simulink model "gnc_simplified"  (R2025b)
settings: Solver=ode2  StartTime=0.0  StopTime=inf  FixedStep=1/100  RelTol=1e-3
undefined symbols (not defined in the file or in its folder): DiscIntNeverNeededParam, dspblkCoreblockFVToolHelper, gcbh
libraries: simulink x5, eeGeneralControl x5
(part 2 of 4)

== system gnc_simplified/INDI/Thrust ==
  note: float32 delta_t
      | float32 t_m
      | float32 t_c
  note: Current thrust
      | lever in [-1,1]
  note: Incremental thrust
      | command in [-1,1]
  note: Total thrust
      | command in [0,1]
  thr_inc : Inport  OutDataTypeStr=single  PortDimensions=1
  act_m : Inport  Port=2  OutDataTypeStr=single  PortDimensions=4
  Bias : Bias  Bias=-1  SaturateOnIntegerOverflow=off
  Bias1 : Bias  Bias=0.5  SaturateOnIntegerOverflow=off
  Constant : Constant  OutDataTypeStr=single
  Constant1 : Constant  Value=-1  OutDataTypeStr=single
  Gain : Gain  Gain=2
  Gain1 : Gain  Gain=0.5
  Gain2 : Gain  Gain=0.5
  Limit_Increment : simulink/Discontinuities/Saturation Dynamic  OutMin=[]  OutMax=[]  OutDataTypeStr=Inherit: Same as second input  OutDataType=fixdt(1, 16)  OutScaling=2^-10  DoSatur=off
  Minus1 : Sum  Inputs=+-
  Minus2 : Sum  Inputs=+-
  Mux : Mux  Inputs=3
  Plus1 : Sum
  Scope : Scope  NumInputPorts=4
      settings: ActiveDisplayYMinimum=-2.22188  ActiveDisplayYMaximum=2.10921
  Selector1 : Selector  InputPortWidth=4  IndexOptions=Index vector (dialog)  Indices=4  OutputSizes=1
  thr_moni : Outport  OutDataTypeStr=single  PortDimensions=3
  thr : Outport  Port=2  OutDataTypeStr=single  PortDimensions=1
  inc_moni : Outport  Port=3
  wires:
  Mux/1 -> thr_moni/1
  Bias/1 -> Scope/1, Mux/2, Minus1/2, Minus2/2, Scope/3, Plus1/2
  Gain/1 -> Bias/1
  Limit_Increment/1 -> Plus1/1, Gain2/1, Scope/2, Mux/1  "thr_inc"
  act_m/1 -> Selector1/1
  Selector1/1 -> Gain/1
  Plus1/1 -> Gain1/1
  Gain1/1 -> Bias1/1
  Bias1/1 -> Scope/4, Mux/3, thr/1
  Gain2/1 -> inc_moni/1
  Constant/1 -> Minus1/1
  thr_inc/1 -> Limit_Increment/2
  Minus1/1 -> Limit_Increment/1
  Minus2/1 -> Limit_Increment/3
  Constant1/1 -> Minus2/1

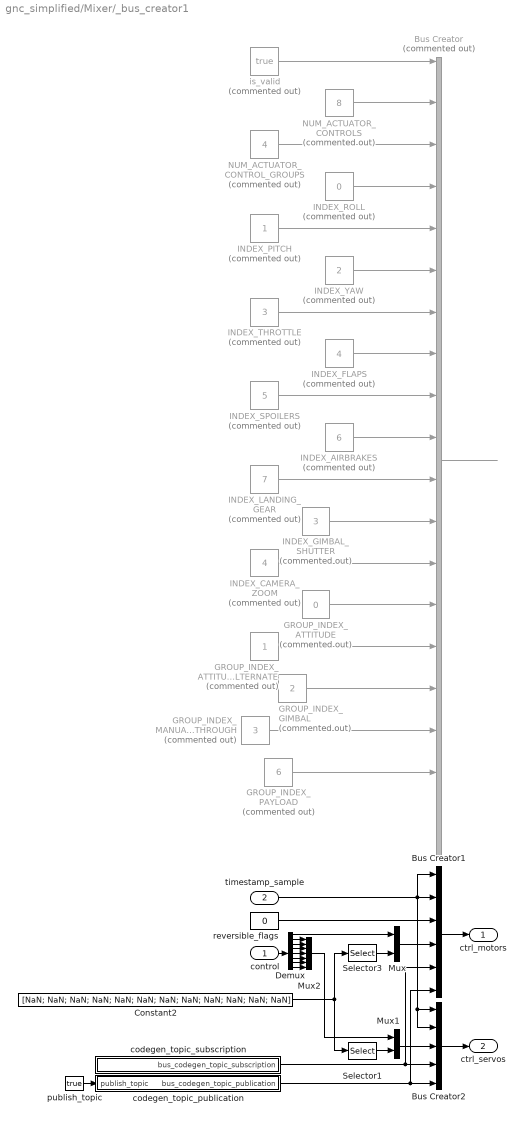
== system gnc_simplified/Mixer/_bus_creator1 ==
  control : Inport  OutDataTypeStr=single  PortDimensions=8
  timestamp_sample : Inport  Port=2  OutDataTypeStr=uint64  PortDimensions=1
  Bus Creator : BusCreator  Commented=on  Inputs=20  OutDataTypeStr=Bus:actuator_controls_0_bus
      settings: InheritFromInputs=off
  Bus Creator1 : BusCreator  Inputs=6  OutDataTypeStr=Bus: IFRCG_Bus_Topic_ActuatorMotors
      settings: InheritFromInputs=off
  Bus Creator2 : BusCreator  Inputs=5  OutDataTypeStr=Bus: IFRCG_Bus_Topic_ActuatorServos
      settings: InheritFromInputs=off
  Constant2 : Constant  Value=[NaN; NaN; NaN; NaN; NaN; NaN; NaN; NaN; NaN; NaN; NaN; NaN]  OutDataTypeStr=single
  Demux : Demux  Outputs=8
  GROUP_INDEX_ATTITUDE : Constant  Commented=on  Value=0  OutDataTypeStr=uint8
  GROUP_INDEX_ATTITUDE_ALTERNATE : Constant  Commented=on  OutDataTypeStr=uint8
  GROUP_INDEX_GIMBAL : Constant  Commented=on  Value=2  OutDataTypeStr=uint8
  GROUP_INDEX_MANUAL_PASSTHROUGH : Constant  Commented=on  Value=3  OutDataTypeStr=uint8
  GROUP_INDEX_PAYLOAD : Constant  Commented=on  Value=6  OutDataTypeStr=uint8
  INDEX_AIRBRAKES : Constant  Commented=on  Value=6  OutDataTypeStr=uint8
  INDEX_CAMERA_ZOOM : Constant  Commented=on  Value=4  OutDataTypeStr=uint8
  INDEX_FLAPS : Constant  Commented=on  Value=4  OutDataTypeStr=uint8
  INDEX_GIMBAL_SHUTTER : Constant  Commented=on  Value=3  OutDataTypeStr=uint8
  INDEX_LANDING_GEAR : Constant  Commented=on  Value=7  OutDataTypeStr=uint8
  INDEX_PITCH : Constant  Commented=on  OutDataTypeStr=uint8
  INDEX_ROLL : Constant  Commented=on  Value=0  OutDataTypeStr=uint8
  INDEX_SPOILERS : Constant  Commented=on  Value=5  OutDataTypeStr=uint8
  INDEX_THROTTLE : Constant  Commented=on  Value=3  OutDataTypeStr=uint8
  INDEX_YAW : Constant  Commented=on  Value=2  OutDataTypeStr=uint8
  Mux : Mux  Inputs=2
  Mux1 : Mux  Inputs=2
  Mux2 : Mux  Inputs=7
  NUM_ACTUATOR_CONTROLS : Constant  Commented=on  Value=8  OutDataTypeStr=uint8
  NUM_ACTUATOR_CONTROL_GROUPS : Constant  Commented=on  Value=4  OutDataTypeStr=uint8
  Selector1 : Selector  InputPortWidth=12  IndexOptions=Index vector (dialog)  Indices=1  OutputSizes=1
  Selector3 : Selector  InputPortWidth=12  IndexOptions=Index vector (dialog)  Indices=1:11  OutputSizes=1
  codegen_topic_publication : Subsystem
  codegen_topic_subscription : Subsystem
  is_valid : Constant  Commented=on  Value=true  OutDataTypeStr=boolean
  publish_topic : Constant  Value=true  OutDataTypeStr=boolean
  reversible_flags : Constant  Value=0  OutDataTypeStr=uint16
  ctrl_motors : Outport  OutDataTypeStr=Bus: IFRCG_Bus_Topic_ActuatorMotors  VectorParamsAs1DForOutWhenUnconnected=off
  ctrl_servos : Outport  Port=2  OutDataTypeStr=Bus: IFRCG_Bus_Topic_ActuatorServos  VectorParamsAs1DForOutWhenUnconnected=off
  wires:
  Bus Creator/1 -> ?
  ? -> Bus Creator/20
  ? -> Bus Creator/19
  GROUP_INDEX_ATTITUDE_ALTERNATE/1 -> Bus Creator/15
  GROUP_INDEX_ATTITUDE/1 -> Bus Creator/14
  INDEX_LANDING_GEAR/1 -> Bus Creator/11
  INDEX_AIRBRAKES/1 -> Bus Creator/10
  INDEX_SPOILERS/1 -> Bus Creator/9
  INDEX_FLAPS/1 -> Bus Creator/8
  INDEX_THROTTLE/1 -> Bus Creator/7
  INDEX_YAW/1 -> Bus Creator/6
  INDEX_PITCH/1 -> Bus Creator/5
  INDEX_ROLL/1 -> Bus Creator/4
  NUM_ACTUATOR_CONTROL_GROUPS/1 -> Bus Creator/3
  NUM_ACTUATOR_CONTROLS/1 -> Bus Creator/2
  is_valid/1 -> Bus Creator/1
  INDEX_GIMBAL_SHUTTER/1 -> Bus Creator/12
  INDEX_CAMERA_ZOOM/1 -> Bus Creator/13
  GROUP_INDEX_GIMBAL/1 -> Bus Creator/16
  GROUP_INDEX_MANUAL_PASSTHROUGH/1 -> Bus Creator/17
  GROUP_INDEX_PAYLOAD/1 -> Bus Creator/18
  Bus Creator1/1 -> ctrl_motors/1
  Bus Creator2/1 -> ctrl_servos/1
  Mux1/1 -> Bus Creator2/3
  timestamp_sample/1 -> Bus Creator2/1, Bus Creator2/2, Bus Creator1/1, Bus Creator1/2
  reversible_flags/1 -> Bus Creator1/3
  publish_topic/1 -> codegen_topic_publication/1(publish_topic)
  codegen_topic_subscription/1(bus_codegen_topic_subscription) -> Bus Creator2/4, Bus Creator1/5
  codegen_topic_publication/1(bus_codegen_topic_publication) -> Bus Creator1/6, Bus Creator2/5
  Selector3/1 -> Mux/2
  Mux/1 -> Bus Creator1/4
  Demux/2 -> Mux2/1
  Demux/3 -> Mux2/2
  Demux/4 -> Mux2/3
  Demux/5 -> Mux2/4
  Demux/6 -> Mux2/5
  Demux/7 -> Mux2/6
  Demux/8 -> Mux2/7
  control/1 -> Demux/1
  Demux/1 -> Mux/1
  Mux2/1 -> Mux1/1
  Selector1/1 -> Mux1/2
  Constant2/1 -> Selector1/1, Selector3/1

== system gnc_simplified/Mixer/_bus_creator2 ==
  control : Inport  OutDataTypeStr=single  PortDimensions=8
  timestamp_sample : Inport  Port=2  OutDataTypeStr=double  PortDimensions=1
  Bus Creator : BusCreator  Inputs=20  OutDataTypeStr=Bus:actuator_controls_0_bus
      settings: InheritFromInputs=off
  GROUP_INDEX_ATTITUDE : Constant  Value=0  OutDataTypeStr=uint8
  GROUP_INDEX_ATTITUDE_ALTERNATE : Constant  OutDataTypeStr=uint8
  GROUP_INDEX_GIMBAL : Constant  Value=2  OutDataTypeStr=uint8
  GROUP_INDEX_MANUAL_PASSTHROUGH : Constant  Value=3  OutDataTypeStr=uint8
  GROUP_INDEX_PAYLOAD : Constant  Value=6  OutDataTypeStr=uint8
  INDEX_AIRBRAKES : Constant  Value=6  OutDataTypeStr=uint8
  INDEX_CAMERA_ZOOM : Constant  Value=4  OutDataTypeStr=uint8
  INDEX_FLAPS : Constant  Value=4  OutDataTypeStr=uint8
  INDEX_GIMBAL_SHUTTER : Constant  Value=3  OutDataTypeStr=uint8
  INDEX_LANDING_GEAR : Constant  Value=7  OutDataTypeStr=uint8
  INDEX_PITCH : Constant  OutDataTypeStr=uint8
  INDEX_ROLL : Constant  Value=0  OutDataTypeStr=uint8
  INDEX_SPOILERS : Constant  Value=5  OutDataTypeStr=uint8
  INDEX_THROTTLE : Constant  Value=3  OutDataTypeStr=uint8
  INDEX_YAW : Constant  Value=2  OutDataTypeStr=uint8
  NUM_ACTUATOR_CONTROLS : Constant  Value=8  OutDataTypeStr=uint8
  NUM_ACTUATOR_CONTROL_GROUPS : Constant  Value=4  OutDataTypeStr=uint8
  is_valid : Constant  Value=true  OutDataTypeStr=boolean
  actuator_controls : Outport  OutDataTypeStr=Bus: IFRCG_Bus_Topic_ActuatorControls1  VectorParamsAs1DForOutWhenUnconnected=off
  wires:
  INDEX_ROLL/1 -> Bus Creator/4
  INDEX_SPOILERS/1 -> Bus Creator/9
  is_valid/1 -> Bus Creator/1
  INDEX_CAMERA_ZOOM/1 -> Bus Creator/13
  control/1 -> Bus Creator/20
  GROUP_INDEX_ATTITUDE_ALTERNATE/1 -> Bus Creator/15
  GROUP_INDEX_GIMBAL/1 -> Bus Creator/16
  INDEX_GIMBAL_SHUTTER/1 -> Bus Creator/12
  INDEX_THROTTLE/1 -> Bus Creator/7
  GROUP_INDEX_ATTITUDE/1 -> Bus Creator/14
  Bus Creator/1 -> actuator_controls/1
  INDEX_PITCH/1 -> Bus Creator/5
  GROUP_INDEX_MANUAL_PASSTHROUGH/1 -> Bus Creator/17
  INDEX_FLAPS/1 -> Bus Creator/8
  INDEX_AIRBRAKES/1 -> Bus Creator/10
  NUM_ACTUATOR_CONTROLS/1 -> Bus Creator/2
  GROUP_INDEX_PAYLOAD/1 -> Bus Creator/18
  timestamp_sample/1 -> Bus Creator/19
  INDEX_YAW/1 -> Bus Creator/6
  NUM_ACTUATOR_CONTROL_GROUPS/1 -> Bus Creator/3
  INDEX_LANDING_GEAR/1 -> Bus Creator/11

== system gnc_simplified/Mixer/bus_generator ==
  In1 : Inport
  Bus Creator : BusCreator  Inputs=7  OutDataTypeStr=Bus: IFRCG_Bus_Topic_MainCtrlAxes
      settings: InheritFromInputs=off
  Demux : Demux
  codegen_topic_publication : Subsystem
  codegen_topic_subscription : Subsystem
  publish_topic : Constant  Value=true  OutDataTypeStr=boolean
  timestamp : Constant  Value=0  OutDataTypeStr=uint64
  main_ctrl_axes : Outport  OutDataTypeStr=Bus: IFRCG_Bus_Topic_MainCtrlAxes
  wires:
  Demux/4 -> Bus Creator/5
  In1/1 -> Demux/1
  Demux/1 -> Bus Creator/2
  Demux/2 -> Bus Creator/3
  Bus Creator/1 -> main_ctrl_axes/1
  timestamp/1 -> Bus Creator/1
  Demux/3 -> Bus Creator/4
  publish_topic/1 -> codegen_topic_publication/1(publish_topic)
  codegen_topic_publication/1(bus_codegen_topic_publication) -> Bus Creator/7
  codegen_topic_subscription/1(bus_codegen_topic_subscription) -> Bus Creator/6

== system gnc_simplified/Modal/Subsystem2 ==
  note: [ Eta    ]
      | [ Delta ]
  mode : Inport
  dx : Inport  Port=2
  u0 : Inport  Port=3
  u : Inport  Port=4
  param : Inport  Port=5
  Constant : Constant  Value=0
  Delay : Delay  DelayLength=1
  Demux : Demux  Outputs=2
  Demux1 : Demux  Outputs=2
  Demux2 : Demux  Outputs=2
  Detect Change : simulink/Logic and Bit Operations/Detect Change  vinit=0  OutDataTypeStr=boolean
  Discrete-Time Integrator : DiscreteIntegrator  ExternalReset=sampled level  InitialConditionSource=external  SampleTime=-1  ShowStatePort=on  ICPrevOutput=DiscIntNeverNeededParam  ICPrevScaledInput=DiscIntNeverNeededParam
  Discrete-Time Integrator1 : DiscreteIntegrator  ExternalReset=sampled level  InitialConditionSource=external  SampleTime=-1  ShowStatePort=on  ICPrevOutput=DiscIntNeverNeededParam  ICPrevScaledInput=DiscIntNeverNeededParam
  MATLAB Function : MATLAB Function  TreatAsAtomicUnit=on
  MATLAB Function1 : MATLAB Function  TreatAsAtomicUnit=on
  Mux : Mux  Inputs=2
  Selector4 : Selector  InputPortWidth=4  IndexOptions=Index vector (dialog)  Indices=[2 4]  OutputSizes=1
  Switch : Switch  Criteria=u2 > Threshold  SaturateOnIntegerOverflow=off  InputSameDT=off
  x : Outport  VectorParamsAs1DForOutWhenUnconnected=off
  wires:
  Constant/1 -> Switch/3
  Detect Change/1 -> Switch/1  "external trigger"
  Delay/1 -> Switch/2
  Selector4/1 -> Demux1/1
  Discrete-Time Integrator1/1 -> Mux/2  "x"
  Mux/1 -> x/1
  Discrete-Time Integrator/1 -> Mux/1
  Demux1/1 -> MATLAB Function/3(u0)
  Demux/2 -> MATLAB Function1/4(u)  "u"
  Demux/1 -> MATLAB Function/4(u)
  Demux1/2 -> MATLAB Function1/3(u0)
  Demux2/2 -> Discrete-Time Integrator1/1
  Demux2/1 -> Discrete-Time Integrator/1
  Discrete-Time Integrator1/State -> MATLAB Function1/1(x)
  dx/1 -> Demux2/1
  u0/1 -> Selector4/1
  MATLAB Function1/1(trigger) -> Discrete-Time Integrator1/2  "general trigger"
  MATLAB Function1/2(x0) -> Discrete-Time Integrator1/3
  Switch/1 -> MATLAB Function1/2(external), MATLAB Function/2(external)  "external trigger"
  Discrete-Time Integrator/State -> MATLAB Function/1(x)
  mode/1 -> Delay/1, Detect Change/1
  MATLAB Function/2(x0) -> Discrete-Time Integrator/3
  MATLAB Function/1(trigger) -> Discrete-Time Integrator/2
  u/1 -> Demux/1
  param/1 -> MATLAB Function/5(param), MATLAB Function1/5(param)

== system gnc_simplified/Subsystem/Actuator_Model ==
  rc_channel : Inport
  main_axes : Inport  Port=2  OutDataTypeStr=Bus: IFRCG_Bus_Topic_MainCtrlAxes
  act_lims : Inport  Port=3
  Actuator Model : Subsystem
  Subsystem1 : Subsystem
  act_m : Outport
  rc_mode : Outport  Port=2  OutDataTypeStr=uint8
  rc_trim : Outport  Port=3  PortDimensions=4
  wires:
  rc_channel/1 -> Subsystem1/1(RC_channels)
  Subsystem1/3(Safety_Switch) -> Actuator Model/2(Safety_Switch)
  Subsystem1/2(RC_controls) -> rc_trim/1, Actuator Model/1(RC_controls)
  Actuator Model/1(Delayed) -> act_m/1
  main_axes/1 -> Actuator Model/3(AP_controls)
  act_lims/1 -> Actuator Model/4(act_lims)
  Subsystem1/1(rc_mode) -> rc_mode/1

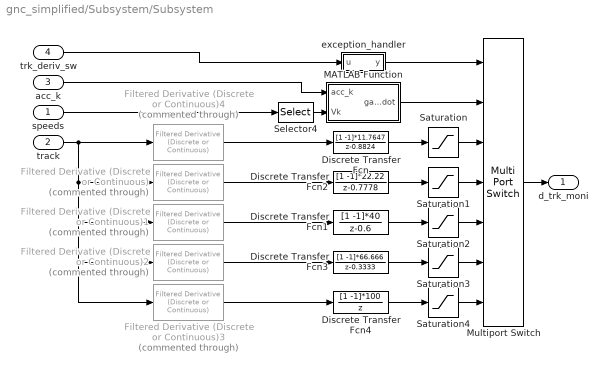
== system gnc_simplified/Subsystem/Subsystem ==
  speeds : Inport
  track : Inport  Port=2
  acc_k : Inport  Port=3
  trk_deriv_sw : Inport  Port=4
  Discrete Transfer Fcn : DiscreteTransferFcn  LoadFcn=dspblkCoreblockFVToolHelper(gcbh,'load');  Numerator=[1 -1]*11.7647  Denominator=[1 -0.8824]
      settings: CopyFcn=dspblkCoreblockFVToolHelper(gcbh,'copy');  DeleteFcn=dspblkCoreblockFVToolHelper(gcbh,'close');  ModelCloseFcn=dspblkCoreblockFVToolHelper(gcbh,'close');  PreSaveFcn=dspblkCoreblockFVToolHelper(gcbh,'presave');  PostSaveFcn=dspblkCoreblockFVToolHelper(gcbh,'postsave');  CloseFcn=dspblkCoreblockFVToolHelper(gcbh,'close');
  Discrete Transfer Fcn1 : DiscreteTransferFcn  LoadFcn=dspblkCoreblockFVToolHelper(gcbh,'load');  Numerator=[1 -1]*40  Denominator=[1 -0.6]
      settings: CopyFcn=dspblkCoreblockFVToolHelper(gcbh,'copy');  DeleteFcn=dspblkCoreblockFVToolHelper(gcbh,'close');  ModelCloseFcn=dspblkCoreblockFVToolHelper(gcbh,'close');  PreSaveFcn=dspblkCoreblockFVToolHelper(gcbh,'presave');  PostSaveFcn=dspblkCoreblockFVToolHelper(gcbh,'postsave');  CloseFcn=dspblkCoreblockFVToolHelper(gcbh,'close');
  Discrete Transfer Fcn2 : DiscreteTransferFcn  LoadFcn=dspblkCoreblockFVToolHelper(gcbh,'load');  Numerator=[1 -1]*22.22  Denominator=[1 -0.7778]
      settings: CopyFcn=dspblkCoreblockFVToolHelper(gcbh,'copy');  DeleteFcn=dspblkCoreblockFVToolHelper(gcbh,'close');  ModelCloseFcn=dspblkCoreblockFVToolHelper(gcbh,'close');  PreSaveFcn=dspblkCoreblockFVToolHelper(gcbh,'presave');  PostSaveFcn=dspblkCoreblockFVToolHelper(gcbh,'postsave');  CloseFcn=dspblkCoreblockFVToolHelper(gcbh,'close');
  Discrete Transfer Fcn3 : DiscreteTransferFcn  LoadFcn=dspblkCoreblockFVToolHelper(gcbh,'load');  Numerator=[1 -1]*66.666  Denominator=[1 -0.3333]
      settings: CopyFcn=dspblkCoreblockFVToolHelper(gcbh,'copy');  DeleteFcn=dspblkCoreblockFVToolHelper(gcbh,'close');  ModelCloseFcn=dspblkCoreblockFVToolHelper(gcbh,'close');  PreSaveFcn=dspblkCoreblockFVToolHelper(gcbh,'presave');  PostSaveFcn=dspblkCoreblockFVToolHelper(gcbh,'postsave');  CloseFcn=dspblkCoreblockFVToolHelper(gcbh,'close');
  Discrete Transfer Fcn4 : DiscreteTransferFcn  LoadFcn=dspblkCoreblockFVToolHelper(gcbh,'load');  Numerator=[1 -1]*100  Denominator=[1 0]
      settings: CopyFcn=dspblkCoreblockFVToolHelper(gcbh,'copy');  DeleteFcn=dspblkCoreblockFVToolHelper(gcbh,'close');  ModelCloseFcn=dspblkCoreblockFVToolHelper(gcbh,'close');  PreSaveFcn=dspblkCoreblockFVToolHelper(gcbh,'presave');  PostSaveFcn=dspblkCoreblockFVToolHelper(gcbh,'postsave');  CloseFcn=dspblkCoreblockFVToolHelper(gcbh,'close');
  Filtered Derivative (Discrete or Continuous) : eeGeneralControl/Filtered Derivative (Discrete or Continuous)  Commented=through  K=1  T=0.04  B=inf  A=-inf  minRatio=10  init_option=Inherited from block input  x0=0  Ts=-1
      settings: LibrarySourceBlock=|
      | ee_sl_lib/General Control/Filtered Derivative
      | (Discrete or Continuous)
  Filtered Derivative (Discrete or Continuous)1 : eeGeneralControl/Filtered Derivative (Discrete or Continuous)  Commented=through  K=1  T=0.02  B=inf  A=-inf  minRatio=10  init_option=Inherited from block input  x0=0  Ts=-1
      settings: LibrarySourceBlock=|
      | ee_sl_lib/General Control/Filtered Derivative
      | (Discrete or Continuous)
  Filtered Derivative (Discrete or Continuous)2 : eeGeneralControl/Filtered Derivative (Discrete or Continuous)  Commented=through  K=1  T=0.01  B=inf  A=-inf  minRatio=10  init_option=Inherited from block input  x0=0  Ts=-1
      settings: LibrarySourceBlock=|
      | ee_sl_lib/General Control/Filtered Derivative
      | (Discrete or Continuous)
  Filtered Derivative (Discrete or Continuous)3 : eeGeneralControl/Filtered Derivative (Discrete or Continuous)  Commented=through  K=1  T=0.005  B=inf  A=-inf  minRatio=10  init_option=Inherited from block input  x0=0  Ts=-1
      settings: LibrarySourceBlock=|
      | ee_sl_lib/General Control/Filtered Derivative
      | (Discrete or Continuous)
  Filtered Derivative (Discrete or Continuous)4 : eeGeneralControl/Filtered Derivative (Discrete or Continuous)  Commented=through  K=1  T=0.08  B=inf  A=-inf  minRatio=10  init_option=Inherited from block input  x0=0  Ts=-1
      settings: LibrarySourceBlock=|
      | ee_sl_lib/General Control/Filtered Derivative
      | (Discrete or Continuous)
  MATLAB Function : MATLAB Function  TreatAsAtomicUnit=on
  Multiport Switch : MultiPortSwitch  Inputs=6  SaturateOnIntegerOverflow=off  InputSameDT=off
  Saturation{,1..4} (5 alike) : Saturate  UpperLimit=pi  LowerLimit=-pi
  Selector4 : Selector  InputPortWidth=2  IndexOptions=Index vector (dialog)  Indices=1  OutputSizes=1
  exception_handler : MATLAB Function  TreatAsAtomicUnit=on
  d_trk_moni : Outport  PortDimensions=2
  wires:
  Multiport Switch/1 -> d_trk_moni/1
  trk_deriv_sw/1 -> exception_handler/1(u)
  Saturation3/1 -> Multiport Switch/6
  Filtered Derivative (Discrete or Continuous)3/1 -> Discrete Transfer Fcn4/1
  Saturation2/1 -> Multiport Switch/5
  Filtered Derivative (Discrete or Continuous)2/1 -> Discrete Transfer Fcn3/1
  Discrete Transfer Fcn3/1 -> Saturation3/1
  Selector4/1 -> MATLAB Function/2(Vk)
  Discrete Transfer Fcn/1 -> Saturation/1
  Discrete Transfer Fcn2/1 -> Saturation1/1
  Saturation4/1 -> Multiport Switch/7
  Discrete Transfer Fcn4/1 -> Saturation4/1
  Filtered Derivative (Discrete or Continuous)1/1 -> Discrete Transfer Fcn1/1
  track/1 -> Filtered Derivative (Discrete or Continuous)3/1, Filtered Derivative (Discrete or Continuous)2/1, Filtered Derivative (Discrete or Continuous)1/1, Filtered Derivative (Discrete or Continuous)/1, Filtered Derivative (Discrete or Continuous)4/1
  Filtered Derivative (Discrete or Continuous)/1 -> Discrete Transfer Fcn2/1
  acc_k/1 -> MATLAB Function/1(acc_k)
  Filtered Derivative (Discrete or Continuous)4/1 -> Discrete Transfer Fcn/1
  Saturation1/1 -> Multiport Switch/4
  MATLAB Function/1(gachi_dot) -> Multiport Switch/2
  Discrete Transfer Fcn1/1 -> Saturation2/1
  Saturation/1 -> Multiport Switch/3
  speeds/1 -> Selector4/1
  exception_handler/1(y) -> Multiport Switch/1

== system gnc_simplified/Subsystem/Subsystem1 ==
  acc_g_vlp : Inport
  acc_g_filt : Inport  Port=2
  Bus Creator : BusCreator  Inputs=5  OutDataTypeStr=Bus: IFRCG_Bus_Topic_AccelMonitor
      settings: InheritFromInputs=off
  codegen_topic_publication : Subsystem
  codegen_topic_subscription : Subsystem
  publish_topic : Constant  Value=true  OutDataTypeStr=boolean
  timestamp : Constant  Value=0  OutDataTypeStr=uint64
  acc_moni : Outport  OutDataTypeStr=Bus: IFRCG_Bus_Topic_AccelMonitor
  wires:
  acc_g_filt/1 -> Bus Creator/3
  acc_g_vlp/1 -> Bus Creator/2
  codegen_topic_publication/1(bus_codegen_topic_publication) -> Bus Creator/5
  codegen_topic_subscription/1(bus_codegen_topic_subscription) -> Bus Creator/4
  publish_topic/1 -> codegen_topic_publication/1(publish_topic)
  timestamp/1 -> Bus Creator/1
  Bus Creator/1 -> acc_moni/1

== system gnc_simplified/Subsystem/Subsystem2 ==
  track_deriv : Inport  OutDataTypeStr=Bus: IFRCG_Bus_Topic_TrackDerivMonitor
  trk_deriv_sw : Inport  Port=2
  Bus Selector : BusSelector  OutputSignals=gamma_dot_acc,chi_dot_acc,gamma_dot_der_008,chi_dot_der_008,gamma_dot_der_004,chi_dot_der_004,gamma_dot_der_002,chi_dot_der_002,gamma_dot_der_001,chi_dot_der_001,gamma_dot_der_0005,chi_dot_der_0005
  Multiport Switch : MultiPortSwitch  Inputs=6  SaturateOnIntegerOverflow=off  InputSameDT=off
  Mux{2,4..8} (6 alike) : Mux  Inputs=2
  exception_handler : MATLAB Function  TreatAsAtomicUnit=on
  trk_deriv : Outport  PortDimensions=2
  wires:
  Mux6/1 -> Multiport Switch/5
  Mux2/1 -> Multiport Switch/6
  Bus Selector/8 -> Mux6/2  "<chi_dot_der_002>"
  Bus Selector/9 -> Mux2/1  "<gamma_dot_der_001>"
  Mux5/1 -> Multiport Switch/4
  Bus Selector/7 -> Mux6/1  "<gamma_dot_der_002>"
  Mux8/1 -> Multiport Switch/3
  Bus Selector/10 -> Mux2/2  "<chi_dot_der_001>"
  Bus Selector/11 -> Mux4/1  "<gamma_dot_der_0005>"
  Bus Selector/3 -> Mux8/1  "<gamma_dot_der_008>"
  Mux7/1 -> Multiport Switch/2
  trk_deriv_sw/1 -> exception_handler/1(u)
  Bus Selector/12 -> Mux4/2  "<chi_dot_der_0005>"
  Bus Selector/5 -> Mux5/1  "<gamma_dot_der_004>"
  Bus Selector/1 -> Mux7/1  "<gamma_dot_acc>"
  track_deriv/1 -> Bus Selector/1
  Bus Selector/4 -> Mux8/2  "<chi_dot_der_008>"
  Multiport Switch/1 -> trk_deriv/1
  Bus Selector/6 -> Mux5/2  "<chi_dot_der_004>"
  Mux4/1 -> Multiport Switch/7
  Bus Selector/2 -> Mux7/2  "<chi_dot_acc>"
  exception_handler/1(y) -> Multiport Switch/1

== system gnc_simplified/Subsystem/Subsystem3 ==
  rc_in : Inport  OutDataTypeStr=Bus: IFRCG_Bus_Topic_RcTrim
  Bus Selector2 : BusSelector  OutputSignals=aileron,elevator,rudder,thrust
  Mux2 : Mux
  rc_controls : Outport  PortDimensions=4
  wires:
  Mux2/1 -> rc_controls/1
  rc_in/1 -> Bus Selector2/1
  Bus Selector2/4 -> Mux2/4  "<thrust>"
  Bus Selector2/1 -> Mux2/1  "<aileron>"
  Bus Selector2/3 -> Mux2/3  "<rudder>"
  Bus Selector2/2 -> Mux2/2  "<elevator>"

== system gnc_simplified/bus_generator/codegen_topic_publication ==
  publish_topic : Inport  OutDataTypeStr=boolean
  Bus_Creator : BusCreator  Inputs=1  OutDataTypeStr=Bus: IFRCG_Bus_CodeGenInternalTopicPublication
      settings: InheritFromInputs=off
  bus_codegen_topic_publication : Outport  OutDataTypeStr=Bus: IFRCG_Bus_CodeGenInternalTopicPublication
  wires:
  publish_topic/1 -> Bus_Creator/1
  Bus_Creator/1 -> bus_codegen_topic_publication/1

== system gnc_simplified/bus_generator/codegen_topic_subscription ==
  Bus_Creator : BusCreator  Inputs=2  OutDataTypeStr=Bus: IFRCG_Bus_CodeGenInternalTopicSubscription
      settings: InheritFromInputs=off
  updated : Constant  Value=false  OutDataTypeStr=boolean
  updated_counter : Constant  Value=0  OutDataTypeStr=uint64
  bus_codegen_topic_subscription : Outport  OutDataTypeStr=Bus: IFRCG_Bus_CodeGenInternalTopicSubscription
  wires:
  Bus_Creator/1 -> bus_codegen_topic_subscription/1
  updated_counter/1 -> Bus_Creator/2
  updated/1 -> Bus_Creator/1

== system gnc_simplified/bus_generator1/codegen_topic_publication ==
  publish_topic : Inport  OutDataTypeStr=boolean
  Bus_Creator : BusCreator  Inputs=1  OutDataTypeStr=Bus: IFRCG_Bus_CodeGenInternalTopicPublication
      settings: InheritFromInputs=off
  bus_codegen_topic_publication : Outport  OutDataTypeStr=Bus: IFRCG_Bus_CodeGenInternalTopicPublication
  wires:
  Bus_Creator/1 -> bus_codegen_topic_publication/1
  publish_topic/1 -> Bus_Creator/1

== system gnc_simplified/bus_generator1/codegen_topic_subscription ==
  Bus_Creator : BusCreator  Inputs=2  OutDataTypeStr=Bus: IFRCG_Bus_CodeGenInternalTopicSubscription
      settings: InheritFromInputs=off
  updated : Constant  Value=false  OutDataTypeStr=boolean
  updated_counter : Constant  Value=0  OutDataTypeStr=uint64
  bus_codegen_topic_subscription : Outport  OutDataTypeStr=Bus: IFRCG_Bus_CodeGenInternalTopicSubscription
  wires:
  updated/1 -> Bus_Creator/1
  updated_counter/1 -> Bus_Creator/2
  Bus_Creator/1 -> bus_codegen_topic_subscription/1

== system gnc_simplified/INDI/Attitude/Nonlinear_inversion ==
  d/dt_att_c : Inport
  param : Inport  Port=2  OutDataTypeStr=Bus: IFRCG_Bus_Params_Gnc
  att_m : Inport  Port=3
  d/dt_gachiv_m : Inport  Port=4  OutDataTypeStr=single  PortDimensions=3
  path_m : Inport  Port=5
  Limit_command : MATLAB Function  TreatAsAtomicUnit=on
  Rate_Command_Generator : MATLAB Function  TreatAsAtomicUnit=on
  Selector : Selector  InputPortWidth=2  IndexOptions=Index vector (dialog)  Indices=1  OutputSizes=1
  rates_ltd : Outport
  wires:
  path_m/1 -> Selector/1
  Selector/1 -> Rate_Command_Generator/3(gamma_m)
  att_m/1 -> Rate_Command_Generator/4(att_m)
  Rate_Command_Generator/1(pqr_cmd) -> Limit_command/2(pqr_c)
  param/1 -> Limit_command/1(param)
  d/dt_att_c/1 -> Rate_Command_Generator/1(att_dot_cmd)
  d/dt_gachiv_m/1 -> Rate_Command_Generator/2(gachiv_dot_m)
  Limit_command/1(rates_ltd) -> rates_ltd/1

== system gnc_simplified/INDI/Attitude/Pseudo-control ==
  note: float32[5] att_cmd
      | float32[5] att_m
      | float32[5] att_err
      | float32[5] att_dot_cmd
  note: Control error
  note: Control gain
  att_c : Inport  OutDataTypeStr=single  PortDimensions=5
  roll_lim : Inport  Port=2  OutDataTypeStr=single  PortDimensions=1
  att_m : Inport  Port=3  OutDataTypeStr=single  PortDimensions=5
  param : Inport  Port=4  OutDataTypeStr=Bus: IFRCG_Bus_Params_Gnc
  Bus Creator : BusCreator  Inputs=4
  Bus Selector : BusSelector  OutputSignals=Ifr_Gnc.I_K_ATT_ALP,Ifr_Gnc.I_K_ATT_THE,Ifr_Gnc.I_K_ATT_BET,Ifr_Gnc.I_K_ATT_PSI,Ifr_Gnc.I_K_ATT_PHI
  Gain{,2..4,11..12} (6 alike) : Gain  Gain=180/pi*ones(5,1)
  Limit_angles : MATLAB Function  TreatAsAtomicUnit=on
  Mux1 : Mux  Inputs=5
  Product2 : Product
  Scope : Scope  NumInputPorts=2
      settings: ActiveDisplayYMinimum=-1206.3319816589355  ActiveDisplayYMaximum=675.23673629760742  DataLoggingVariableName=ScopeData3
  Scope1 : Scope  NumInputPorts=4
      settings: ActiveDisplayYMinimum=-56.25  ActiveDisplayYMaximum=56.25
  Sum1 : Sum  Inputs=-+|
  att_moni : Outport  OutDataTypeStr=single  PortDimensions=20
  d/dt_att_c : Outport  Port=2  OutDataTypeStr=single  PortDimensions=5
  wires:
  Mux1/1 -> Product2/1
  att_c/1 -> Gain3/1, Limit_angles/2(att_c)
  Product2/1 -> Gain/1, d/dt_att_c/1
  Bus Selector/3 -> Mux1/3  "<I_K_ATT_BET>"
  Bus Selector/1 -> Mux1/1  "<I_K_ATT_ALP>"
  Bus Selector/4 -> Mux1/4  "<I_K_ATT_PSI>"
  Bus Selector/2 -> Mux1/2  "<I_K_ATT_THE>"
  Bus Selector/5 -> Mux1/5  "<I_K_ATT_PHI>"
  Limit_angles/1(ltd) -> Sum1/2, Gain2/1
  Gain/1 -> Bus Creator/4, Scope/1
  Gain2/1 -> Scope1/2
  Gain3/1 -> Bus Creator/1, Scope1/3
  Gain4/1 -> Bus Creator/2, Scope1/4
  Bus Creator/1 -> att_moni/1
  Sum1/1 -> Gain12/1, Gain11/1, Product2/2
  att_m/1 -> Gain4/1, Sum1/1
  Gain12/1 -> Bus Creator/3, Scope/2
  Gain11/1 -> Scope1/1
  roll_lim/1 -> Limit_angles/3(roll_limit)
  param/1 -> Limit_angles/1(params), Bus Selector/1

== system gnc_simplified/INDI/Monitor/codegen_topic_publication ==
  publish_topic : Inport  OutDataTypeStr=boolean
  Bus_Creator : BusCreator  Inputs=1  OutDataTypeStr=Bus: IFRCG_Bus_CodeGenInternalTopicPublication
      settings: InheritFromInputs=off
  bus_codegen_topic_publication : Outport  OutDataTypeStr=Bus: IFRCG_Bus_CodeGenInternalTopicPublication
  wires:
  publish_topic/1 -> Bus_Creator/1
  Bus_Creator/1 -> bus_codegen_topic_publication/1

== system gnc_simplified/INDI/Monitor/codegen_topic_subscription ==
  Bus_Creator : BusCreator  Inputs=2  OutDataTypeStr=Bus: IFRCG_Bus_CodeGenInternalTopicSubscription
      settings: InheritFromInputs=off
  updated : Constant  Value=false  OutDataTypeStr=boolean
  updated_counter : Constant  Value=0  OutDataTypeStr=uint64
  bus_codegen_topic_subscription : Outport  OutDataTypeStr=Bus: IFRCG_Bus_CodeGenInternalTopicSubscription
  wires:
  Bus_Creator/1 -> bus_codegen_topic_subscription/1
  updated_counter/1 -> Bus_Creator/2
  updated/1 -> Bus_Creator/1

== system gnc_simplified/INDI/Path/Incremental_inversion ==
  note: [alpha,theta,beta,psi,mu]
  d/dt_gachiv_e : Inport
  params : Inport  Port=2  OutDataTypeStr=Bus: IFRCG_Bus_Params_Gnc
  gachiv_m : Inport  Port=3  OutDataTypeStr=single  PortDimensions=3
  abmu_m : Inport  Port=4
  q_dyn : Inport  Port=5
  Attitude_Command_Generator : MATLAB Function  TreatAsAtomicUnit=on
  Constant : Constant  Value=0  OutDataTypeStr=single
  Demux1 : Demux  Outputs=3
  Demux2 : Demux  Outputs=2
  Demux5 : Demux  Outputs=3
  Gain10 : Gain  Gain=180/pi
  Gain9 : Gain  Gain=[180/pi,180/pi,1]
  Minus2 : Sum  Inputs=+-
  Mux : Mux  Inputs=2
  Mux1 : Mux  Inputs=2
  Mux12 : Mux  Inputs=5
  Plus : Sum
  Scope2 : Scope  NumInputPorts=3
      settings: ActiveDisplayYMinimum=-0.066928728080398514  ActiveDisplayYMaximum=0.84679823333079618
  Scope6 : Scope  NumInputPorts=2
      settings: ActiveDisplayYMinimum=-54.584307008348048  ActiveDisplayYMaximum=22.013184027047203  DataLoggingVariableName=ScopeData16
  Selector : Selector  InputPortWidth=3  IndexOptions=Index vector (dialog)  Indices=[1,3]  OutputSizes=1
  angles_c : Outport  OutDataTypeStr=single  PortDimensions=5
  inc_cmd : Outport  Port=2  OutDataTypeStr=single  PortDimensions=3
  wires:
  q_dyn/1 -> Attitude_Command_Generator/5(q_dyn)
  Gain10/1 -> Scope6/2
  Gain9/1 -> Scope6/1
  Attitude_Command_Generator/1(att_inc_reciprocal) -> inc_cmd/1, Demux5/1, Scope2/3, Minus2/2
  Minus2/1 -> Scope2/1
  Attitude_Command_Generator/2(att_inc_inversion) -> Minus2/1, Scope2/2
  Selector/1 -> Attitude_Command_Generator/4(gav_m)
  gachiv_m/1 -> Selector/1
  d/dt_gachiv_e/1 -> Gain9/1, Attitude_Command_Generator/1(gachiv_dot_e)
  abmu_m/1 -> Demux1/1, Attitude_Command_Generator/2(abmu_m)
  Mux12/1 -> Gain10/1, angles_c/1
  params/1 -> Attitude_Command_Generator/3(params)
  Constant/1 -> Mux12/2, Mux12/4, Mux12/3
  Demux2/2 -> Mux12/5
  Demux5/2 -> Mux/2
  Demux5/1 -> Mux/1
  Mux/1 -> Plus/2
  Mux1/1 -> Plus/1
  Demux1/1 -> Mux1/1
  Demux1/3 -> Mux1/2
  Demux2/1 -> Mux12/1
  Plus/1 -> Demux2/1

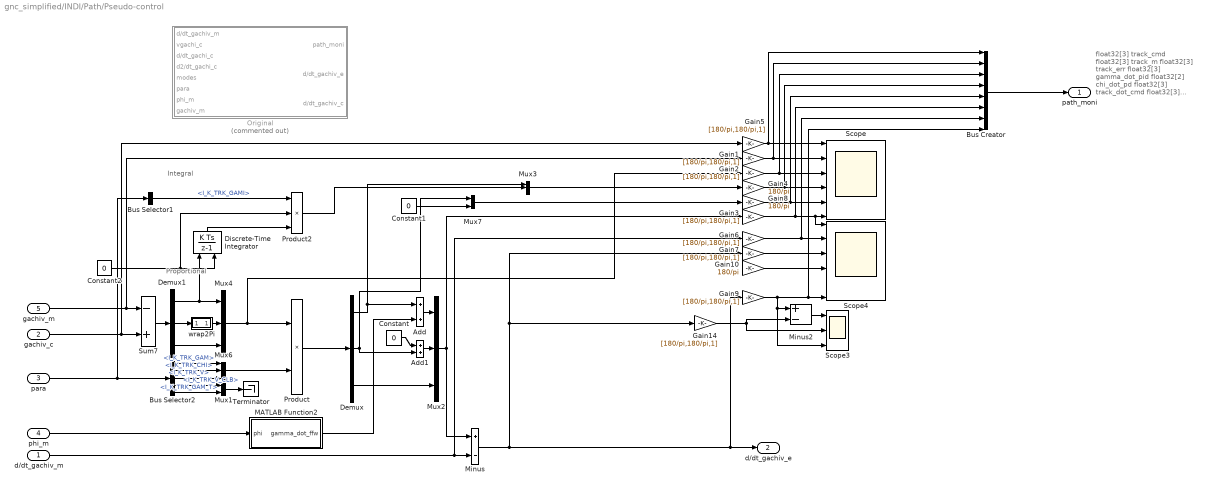
== system gnc_simplified/INDI/Path/Pseudo-control ==
  note: Proportional
  note: Integral
  note: float32[3] track_cmd
      | float32[3] track_m
      | float32[3] track_err
      | float32[3] gamma_dot_pid
      | float32[2] chi_dot_pd
      | float32[3] track_dot_cmd
      | float32[3] track_dot_m
      | float32[3] track_dot_err
  d/dt_gachiv_m : Inport  PortDimensions=3
  gachiv_c : Inport  Port=2
  para : Inport  Port=3  OutDataTypeStr=Bus: IFRCG_Bus_Params_Gnc
  phi_m : Inport  Port=4
  gachiv_m : Inport  Port=5  PortDimensions=3
  Add : Sum
  Add1 : Sum
  Bus Creator : BusCreator  Inputs=8
  Bus Selector1 : BusSelector  OutputSignals=Ifr_Gnc.I_K_TRK_GAMI
  Bus Selector2 : BusSelector  OutputSignals=Ifr_Gnc.I_K_TRK_GAM,Ifr_Gnc.I_K_TRK_CHI,Ifr_Gnc.I_K_TRK_V,Ifr_Gnc.I_K_TRK_V_CLB,Ifr_Gnc.I_K_TRK_GAM_T
  Constant : Constant  Value=0  OutDataTypeStr=single
  Constant1 : Constant  Value=0  OutDataTypeStr=single
  Constant2 : Constant  Value=0  OutDataTypeStr=boolean
  Demux : Demux  Outputs=3
  Demux1 : Demux  Outputs=3
  Discrete-Time Integrator : DiscreteIntegrator  ExternalReset=rising  SampleTime=-1  LimitOutput=on  UpperSaturationLimit=1  LowerSaturationLimit=-1  ICPrevOutput=DiscIntNeverNeededParam  ICPrevScaledInput=DiscIntNeverNeededParam
  Gain{1..3,5..7,9,14} (8 alike) : Gain  Gain=[180/pi,180/pi,1]
  Gain10 : Gain  Gain=180/pi
  Gain4 : Gain  Gain=180/pi
  Gain8 : Gain  Gain=180/pi
  MATLAB Function2 : MATLAB Function  TreatAsAtomicUnit=on
  Minus : Sum  Inputs=+-
  Minus2 : Sum  Inputs=+-
  Mux1 : Mux  Inputs=2
  Mux{2..4,6} (4 alike) : Mux  Inputs=3
  Mux7 : Mux  Inputs=2
  Original : Subsystem  Commented=on
  Product : Product
  Product2 : Product  Inputs=3
  Scope : Scope  NumInputPorts=6
      settings: ActiveDisplayYMinimum=-16.802744671150492  ActiveDisplayYMaximum=22.227899957586231
  Scope3 : Scope  NumInputPorts=3
  Scope4 : Scope  NumInputPorts=6
      settings: ActiveDisplayYMinimum=-20.488040447235107  ActiveDisplayYMaximum=15.403716564178467  DataLoggingVariableName=ScopeData11
  Sum7 : Sum  Inputs=-+
  Terminator : Terminator
  wrap2Pi : Subsystem
  path_moni : Outport
  d/dt_gachiv_e : Outport  Port=2  PortDimensions=3
  wires:
  phi_m/1 -> MATLAB Function2/1(phi)
  para/1 -> Bus Selector1/1, Bus Selector2/1
  Add/1 -> Mux2/1
  Sum7/1 -> Demux1/1
  Mux2/1 -> Minus/1, Gain3/1
  Bus Selector1/1 -> Product2/1  "<I_K_TRK_GAMI>"
  gachiv_m/1 -> Sum7/1, Gain1/1
  Demux/1 -> Add/1, Mux3/1
  Add1/1 -> Mux2/2
  MATLAB Function2/1(gamma_dot_ffw) -> Add/2
  Demux/3 -> Mux2/3
  Gain7/1 -> Scope4/3
  d/dt_gachiv_m/1 -> Minus/2, Gain6/1
  Demux1/2 -> wrap2Pi/1(In1)
  wrap2Pi/1(Out1) -> Mux4/2
  Demux1/3 -> Mux4/3
  Demux1/1 -> Mux4/1, Discrete-Time Integrator/1
  Bus Selector2/1 -> Mux6/1  "<I_K_TRK_GAM>"
  Bus Selector2/2 -> Mux6/2  "<I_K_TRK_CHI>"
  Bus Selector2/3 -> Mux6/3  "<I_K_TRK_V>"
  Mux3/1 -> Gain4/1
  Mux7/1 -> Gain8/1
  Minus/1 -> Gain14/1, Gain7/1, Gain9/1, d/dt_gachiv_e/1
  Gain10/1 -> Scope4/4
  Gain14/1 -> Minus2/2, Scope3/2
  Minus2/1 -> Scope3/1
  gachiv_c/1 -> Sum7/2, Gain5/1
  Gain5/1 -> Bus Creator/1, Scope/1
  Gain1/1 -> Bus Creator/2, Scope/2
  Gain2/1 -> Bus Creator/3, Scope/3
  Gain4/1 -> Bus Creator/4, Scope/4
  Gain3/1 -> Bus Creator/6, Scope4/1, Scope/6
  Gain6/1 -> Bus Creator/7, Scope4/2
  Gain9/1 -> Bus Creator/8, Scope4/6, Minus2/1, Scope3/3
  Gain8/1 -> Bus Creator/5, Scope/5
  Bus Creator/1 -> path_moni/1
  Mux6/1 -> Product/2
  Constant2/1 -> Product2/2, Discrete-Time Integrator/2
  Discrete-Time Integrator/1 -> Product2/3
  Product/1 -> Demux/1
  Demux/2 -> Mux7/1, Add1/2
  Constant/1 -> Add1/1
  Product2/1 -> Mux3/2
  Constant1/1 -> Mux7/2
  Mux4/1 -> Gain2/1, Product/1
  Bus Selector2/5 -> Mux1/2  "<I_K_TRK_GAM_T>"
  Bus Selector2/4 -> Mux1/1  "<I_K_TRK_V_CLB>"
  Mux1/1 -> Terminator/1

== system gnc_simplified/INDI/Rates to surfaces&brakes/Diff and Filter IMU ==
  note: Use filtered derivative of angular velocities from IMU filter module or filter here
  imu_filter : Inport
  act_m : Inport  Port=2
  rates : Inport  Port=3
  params : Inport  Port=4  OutDataTypeStr=Bus: IFRCG_Bus_Params_Gnc
  Bus Selector : BusSelector  OutputSignals=Ifr_Gnc.IMU_FIL_DRTE
  Bus Selector1 : BusSelector  OutputSignals=ang_acc,omega,zeta
  Discrete Transfer Fcn : DiscreteTransferFcn  LoadFcn=dspblkCoreblockFVToolHelper(gcbh,'load');  NumeratorSource=Input port  DenominatorSource=Input port  a0EqualsOne=on
      settings: CopyFcn=dspblkCoreblockFVToolHelper(gcbh,'copy');  DeleteFcn=dspblkCoreblockFVToolHelper(gcbh,'close');  ModelCloseFcn=dspblkCoreblockFVToolHelper(gcbh,'close');  PreSaveFcn=dspblkCoreblockFVToolHelper(gcbh,'presave');  PostSaveFcn=dspblkCoreblockFVToolHelper(gcbh,'postsave');  CloseFcn=dspblkCoreblockFVToolHelper(gcbh,'close');  InputPortMap=u0,p1,p3
  MATLAB Function : MATLAB Function  TreatAsAtomicUnit=on
  Scope : Scope  NumInputPorts=2
      settings: ActiveDisplayYMinimum=-3.8354292782870232  ActiveDisplayYMaximum=3.6294180920878887  DataLoggingVariableName=ScopeData24
  Selector : Selector  InputPortWidth=4  IndexOptions=Index vector (dialog)  Indices=1:3  OutputSizes=1
  Subsystem : Subsystem
  Switch : Switch  Criteria=u2 > Threshold  SaturateOnIntegerOverflow=off  InputSameDT=off
  Switch1 : Switch  Criteria=u2 > Threshold  SaturateOnIntegerOverflow=off  InputSameDT=off
  fromRPAS : Subsystem  Commented=on
  act_del : Outport  OutDataTypeStr=single  PortDimensions=3
  d/dt_pqr_m : Outport  Port=2  OutDataTypeStr=single  PortDimensions=3
  wires:
  act_m/1 -> Selector/1
  Selector/1 -> Subsystem/2(act_m), Discrete Transfer Fcn/1
  MATLAB Function/1(num) -> Discrete Transfer Fcn/2
  MATLAB Function/2(den) -> Discrete Transfer Fcn/3
  imu_filter/1 -> Bus Selector1/1
  rates/1 -> Subsystem/1(rates)
  Switch1/1 -> d/dt_pqr_m/1
  Switch/1 -> act_del/1
  Subsystem/2(act_del) -> Switch/3
  Discrete Transfer Fcn/1 -> Switch/1
  Bus Selector/1 -> Switch/2, Switch1/2  "<IMU_FIL_DRTE>"
  Subsystem/1(dt_pqr_m) -> Switch1/3, Scope/1
  Bus Selector1/1 -> Scope/2, Switch1/1  "<ang_acc>"
  params/1 -> Bus Selector/1
  Bus Selector1/3 -> MATLAB Function/2(zeta)  "<zeta>"
  Bus Selector1/2 -> MATLAB Function/1(omega)  "<omega>"

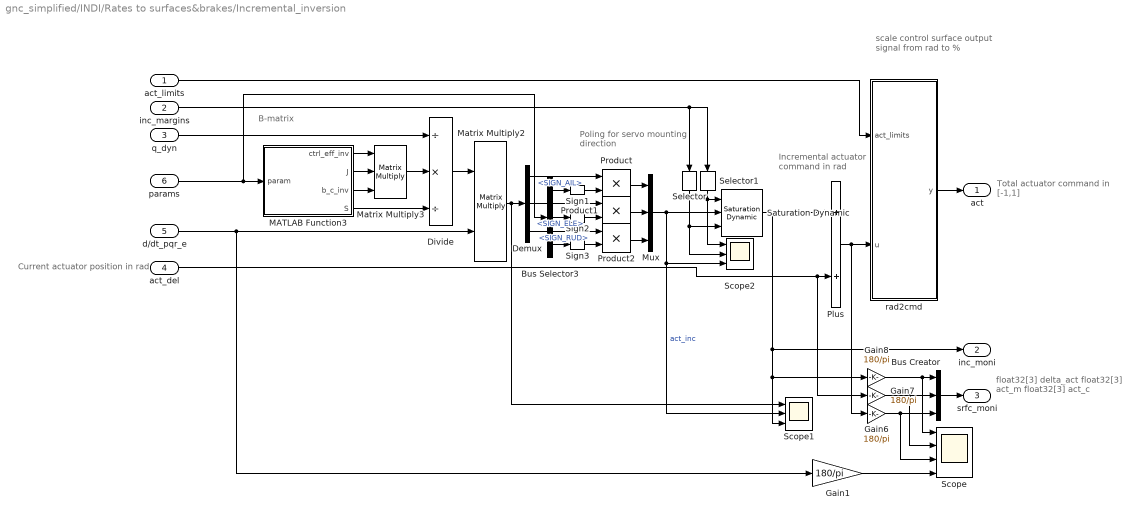
== system gnc_simplified/INDI/Rates to surfaces&brakes/Incremental_inversion ==
  note: B-matrix
  note: float32[3] delta_act
      | float32[3] act_m
      | float32[3] act_c
  note: Incremental
      | actuator
      | command
      | in rad
  note: Current actuator position in rad
  note: scale control
      | surface output
      | signal from
      | rad to %
  note: Total actuator
      | command in [-1,1]
  note: Poling for servo
      | mounting direction
  act_limits : Inport
  inc_margins : Inport  Port=2  OutDataTypeStr=single  PortDimensions=[3,2]
  q_dyn : Inport  Port=3
  act_del : Inport  Port=4  OutDataTypeStr=single  PortDimensions=3
  d/dt_pqr_e : Inport  Port=5
  params : Inport  Port=6  OutDataTypeStr=Bus: IFRCG_Bus_Params_Gnc
  Bus Creator : BusCreator  Inputs=3
  Bus Selector3 : BusSelector  OutputSignals=Ifr_Gnc.SIGN_AIL,Ifr_Gnc.SIGN_ELE,Ifr_Gnc.SIGN_RUD
  Demux : Demux  Outputs=3
  Divide : Product  Inputs=/*/
  Gain{1,6..8} (4 alike) : Gain  Gain=180/pi
  MATLAB Function3 : MATLAB Function  TreatAsAtomicUnit=on
  Matrix Multiply2 : Product  Multiplication=Matrix(*)
  Matrix Multiply3 : Product  Inputs=3  Multiplication=Matrix(*)
  Mux : Mux  Inputs=3
  Plus : Sum
  Product : Product  OutDataTypeStr=single
  Product1 : Product  OutDataTypeStr=single
  Product2 : Product  OutDataTypeStr=single
  Saturation Dynamic : simulink/Discontinuities/Saturation Dynamic  OutMin=[]  OutMax=[]  OutDataTypeStr=Inherit: Same as second input  OutDataType=fixdt(1, 16)  OutScaling=2^-10  DoSatur=off
  Scope : Scope  NumInputPorts=4
      settings: ActiveDisplayYMinimum=-2.1245363890864368  ActiveDisplayYMaximum=1.3972421611797863
  Scope1 : Scope  NumInputPorts=3
      settings: ActiveDisplayYMinimum=-9.9718608856201172  ActiveDisplayYMaximum=9.7918710708618164
  Scope2 : Scope  NumInputPorts=3
      settings: ActiveDisplayYMinimum=-0.59764588236630312  ActiveDisplayYMaximum=0.730759123454152  DataLoggingVariableName=ScopeData21
  Selector : Selector  NumberOfDimensions=2  InputPortWidth=3  IndexOptions=Index vector (dialog),Index vector (dialog)  Indices=1:3,1  OutputSizes=1,1
  Selector1 : Selector  NumberOfDimensions=2  InputPortWidth=3  IndexOptions=Index vector (dialog),Index vector (dialog)  Indices=1:3,2  OutputSizes=1,1
  Sign1 : Signum
  Sign2 : Signum
  Sign3 : Signum
  rad2cmd : MATLAB Function  TreatAsAtomicUnit=on
  act : Outport
  inc_moni : Outport  Port=2
  srfc_moni : Outport  Port=3  OutDataTypeStr=single  PortDimensions=9
  wires:
  Matrix Multiply2/1 -> Scope1/1, Demux/1
  Mux/1 -> Scope1/2, Scope2/3, Saturation Dynamic/2  "act_inc"
  act_del/1 -> Gain7/1, Plus/2
  Plus/1 -> Gain6/1, rad2cmd/2(u)
  Saturation Dynamic/1 -> Gain8/1, Scope1/3, inc_moni/1, Plus/1
  rad2cmd/1(y) -> act/1
  MATLAB Function3/3(b_c_inv) -> Matrix Multiply3/3
  MATLAB Function3/1(ctrl_eff_inv) -> Matrix Multiply3/1
  MATLAB Function3/2(J) -> Matrix Multiply3/2
  d/dt_pqr_e/1 -> Matrix Multiply2/2, Gain1/1
  Matrix Multiply3/1 -> Divide/2
  MATLAB Function3/4(S) -> Divide/3
  Divide/1 -> Matrix Multiply2/1
  Bus Creator/1 -> srfc_moni/1
  Gain1/1 -> Scope/4
  Gain8/1 -> Scope/1, Bus Creator/1
  Gain7/1 -> Bus Creator/2, Scope/2
  Gain6/1 -> Scope/3, Bus Creator/3
  act_limits/1 -> rad2cmd/1(act_limits)
  q_dyn/1 -> Divide/1
  params/1 -> Bus Selector3/1, MATLAB Function3/1(param)
  inc_margins/1 -> Selector/1, Selector1/1
  Selector1/1 -> Scope2/1, Saturation Dynamic/1
  Selector/1 -> Scope2/2, Saturation Dynamic/3
  Demux/2 -> Product1/1
  Bus Selector3/3 -> Sign3/1  "<SIGN_RUD>"
  Bus Selector3/1 -> Sign1/1  "<SIGN_AIL>"
  Demux/1 -> Product/1
  Bus Selector3/2 -> Sign2/1  "<SIGN_ELE>"
  Sign1/1 -> Product/2
  Demux/3 -> Product2/1
  Sign2/1 -> Product1/2
  Sign3/1 -> Product2/2
  Product2/1 -> Mux/3
  Product/1 -> Mux/1
  Product1/1 -> Mux/2

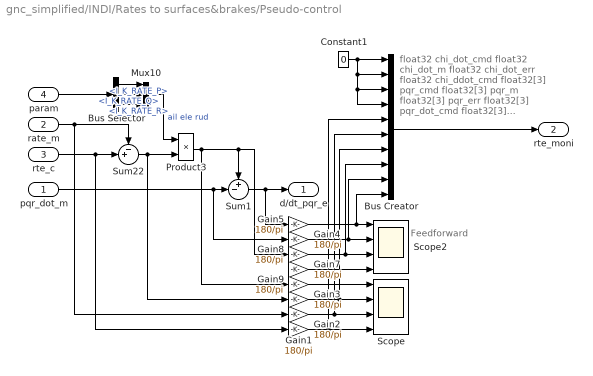
== system gnc_simplified/INDI/Rates to surfaces&brakes/Pseudo-control ==
  note: Feedforward
  note: float32 chi_dot_cmd
      | float32 chi_dot_m
      | float32 chi_dot_err
      | float32 chi_ddot_cmd
      | float32[3] pqr_cmd
      | float32[3] pqr_m
      | float32[3] pqr_err
      | float32[3] pqr_dot_cmd
      | float32[3] pqr_dot_m
      | float32[3] pqr_dot_err
  pqr_dot_m : Inport  OutDataTypeStr=single  PortDimensions=3
  rate_m : Inport  Port=2  OutDataTypeStr=single  PortDimensions=3
  rte_c : Inport  Port=3  OutDataTypeStr=single  PortDimensions=3
  param : Inport  Port=4  OutDataTypeStr=Bus: IFRCG_Bus_Params_Gnc
  Bus Creator : BusCreator  Inputs=10
  Bus Selector : BusSelector  OutputSignals=Ifr_Gnc.I_K_RATE_P,Ifr_Gnc.I_K_RATE_Q,Ifr_Gnc.I_K_RATE_R
  Constant1 : Constant  Value=0  OutDataTypeStr=single
  Gain{1..5,7..9} (8 alike) : Gain  Gain=180/pi
  Mux10 : Mux  Inputs=3
  Product3 : Product
  Scope : Scope  NumInputPorts=4
      settings: ActiveDisplayYMinimum=-53.266675928464281  ActiveDisplayYMaximum=50.598231200988494  DataLoggingVariableName=ScopeData2
  Scope2 : Scope  NumInputPorts=4
      settings: ActiveDisplayYMinimum=-1266.2567672729492  ActiveDisplayYMaximum=2019.7770919799805  DataLoggingVariableName=ScopeData2
  Sum1 : Sum  Inputs=+-|
  Sum22 : Sum  Inputs=-+|
  d/dt_pqr_e : Outport  OutDataTypeStr=single  PortDimensions=3
  rte_moni : Outport  Port=2  OutDataTypeStr=single  PortDimensions=22
  wires:
  Mux10/1 -> Product3/1  "ail ele rud"
  Sum22/1 -> Gain3/1, Product3/2
  rate_m/1 -> Gain1/1, Sum22/1
  param/1 -> Bus Selector/1
  rte_c/1 -> Sum22/2, Gain2/1
  Product3/1 -> Gain8/1, Sum1/1, Gain9/1
  Gain3/1 -> Scope/2, Bus Creator/7
  Gain9/1 -> Scope/1
  Gain8/1 -> Scope2/3, Bus Creator/8
  Gain1/1 -> Scope/3, Bus Creator/6
  Gain2/1 -> Scope/4, Bus Creator/5
  Sum1/1 -> d/dt_pqr_e/1, Gain5/1
  pqr_dot_m/1 -> Gain4/1, Sum1/2
  Gain4/1 -> Scope2/2, Bus Creator/9
  Gain5/1 -> Bus Creator/10, Scope2/1
  Bus Creator/1 -> rte_moni/1
  Gain7/1 -> Scope2/4
  Constant1/1 -> Bus Creator/2, Bus Creator/3, Bus Creator/4, Bus Creator/1
  Bus Selector/1 -> Mux10/1  "<I_K_RATE_P>"
  Bus Selector/2 -> Mux10/2  "<I_K_RATE_Q>"
  Bus Selector/3 -> Mux10/3  "<I_K_RATE_R>"

== system gnc_simplified/Mixer/_bus_creator1/codegen_topic_publication ==
  publish_topic : Inport  OutDataTypeStr=boolean
  Bus_Creator : BusCreator  Inputs=1  OutDataTypeStr=Bus: IFRCG_Bus_CodeGenInternalTopicPublication
      settings: InheritFromInputs=off
  bus_codegen_topic_publication : Outport  OutDataTypeStr=Bus: IFRCG_Bus_CodeGenInternalTopicPublication
  wires:
  publish_topic/1 -> Bus_Creator/1
  Bus_Creator/1 -> bus_codegen_topic_publication/1

== system gnc_simplified/Mixer/_bus_creator1/codegen_topic_subscription ==
  Bus_Creator : BusCreator  Inputs=2  OutDataTypeStr=Bus: IFRCG_Bus_CodeGenInternalTopicSubscription
      settings: InheritFromInputs=off
  updated : Constant  Value=false  OutDataTypeStr=boolean
  updated_counter : Constant  Value=0  OutDataTypeStr=uint64
  bus_codegen_topic_subscription : Outport  OutDataTypeStr=Bus: IFRCG_Bus_CodeGenInternalTopicSubscription
  wires:
  Bus_Creator/1 -> bus_codegen_topic_subscription/1
  updated_counter/1 -> Bus_Creator/2
  updated/1 -> Bus_Creator/1

== system gnc_simplified/Mixer/bus_generator/codegen_topic_publication ==
  publish_topic : Inport  OutDataTypeStr=boolean
  Bus_Creator : BusCreator  Inputs=1  OutDataTypeStr=Bus: IFRCG_Bus_CodeGenInternalTopicPublication
      settings: InheritFromInputs=off
  bus_codegen_topic_publication : Outport  OutDataTypeStr=Bus: IFRCG_Bus_CodeGenInternalTopicPublication
  wires:
  publish_topic/1 -> Bus_Creator/1
  Bus_Creator/1 -> bus_codegen_topic_publication/1

== system gnc_simplified/Mixer/bus_generator/codegen_topic_subscription ==
  Bus_Creator : BusCreator  Inputs=2  OutDataTypeStr=Bus: IFRCG_Bus_CodeGenInternalTopicSubscription
      settings: InheritFromInputs=off
  updated : Constant  Value=false  OutDataTypeStr=boolean
  updated_counter : Constant  Value=0  OutDataTypeStr=uint64
  bus_codegen_topic_subscription : Outport  OutDataTypeStr=Bus: IFRCG_Bus_CodeGenInternalTopicSubscription
  wires:
  Bus_Creator/1 -> bus_codegen_topic_subscription/1
  updated_counter/1 -> Bus_Creator/2
  updated/1 -> Bus_Creator/1

== system gnc_simplified/Subsystem/Actuator_Model/Actuator Model ==
  note: Scale thrust signal
  note: Aileron		[-1, 1]
      | Elevator		[-1, 1]
      | Rudder		[-1, 1]
      | Thrust		[0, 1]
  note: Discrete time thrust
      | dynamics transfer function
      | modelled as PT1 in
      | continuous time (tau = 0.15,
      | ts = 100Hz).
      | See filter_design.m for
      | more details.
  note: Limit
      | between
      | [0,1]
  note: Limit between
      | [-1,1]
  note: Scale actuator
      | signal from
      | % to rad
  note: Current actuator signal in %
      | Thrust [-1, 1]
      | Aileron [-1, 1]
      | Elevator [-1, 1]
      | Rudder [-1, 1]
  note: Current control surface
      | deflection in rad, thrust
      | lever in [0,1].
  note: Actuator model output units need to
      | match increment units of control law.
      | Therefore, controller output must be
      | retransformed to corresponding unit.
  note: Discrete time actuator
      | dynamics transfer function
      | modelled as PT1 in
      | continuous time (tau = 0.05,
      | ts = 100Hz).
      | See filter_design.m for
      | more details.
  RC_controls : Inport
  Safety_Switch : Inport  Port=2
  AP_controls : Inport  Port=3  OutDataTypeStr=Bus: IFRCG_Bus_Topic_MainCtrlAxes
  act_lims : Inport  Port=4
  Bus Selector : BusSelector  OutputSignals=aileron,elevator,rudder,thrust
  Data Type Conversion1 : DataTypeConversion  OutDataTypeStr=single  SaturateOnIntegerOverflow=off  RndMeth=Floor
  Demux : Demux
  MATLAB Function1 : MATLAB Function  TreatAsAtomicUnit=on
  Mux : Mux  Inputs=3
  Mux1 : Mux  Inputs=2
  Mux4 : Mux
  Scope : Scope  NumInputPorts=4
  Scope1 : Scope  NumInputPorts=4
      settings: ActiveDisplayYMinimum=-0.125  ActiveDisplayYMaximum=1.125
  Scope2 : Scope
      settings: ActiveDisplayYMinimum=-1  ActiveDisplayYMaximum=1  DataLoggingVariableName=ScopeData8
  Switch1 : Switch  Criteria=u2 > Threshold  SaturateOnIntegerOverflow=off  InputSameDT=off
  act_alg : DiscreteTransferFcn  Numerator=[0.0909 0.0909]  Denominator=[1 -0.8182]
  act_alg2 : DiscreteTransferFcn  LoadFcn=dspblkCoreblockFVToolHelper(gcbh,'load');  Numerator=[0.0323 0.0323]  Denominator=[1 -0.9355]
      settings: CopyFcn=dspblkCoreblockFVToolHelper(gcbh,'copy');  DeleteFcn=dspblkCoreblockFVToolHelper(gcbh,'close');  ModelCloseFcn=dspblkCoreblockFVToolHelper(gcbh,'close');  PreSaveFcn=dspblkCoreblockFVToolHelper(gcbh,'presave');  PostSaveFcn=dspblkCoreblockFVToolHelper(gcbh,'postsave');  CloseFcn=dspblkCoreblockFVToolHelper(gcbh,'close');
  cmd2deg : MATLAB Function  TreatAsAtomicUnit=on
  limit control output : MATLAB Function  TreatAsAtomicUnit=on
  limit control output3 : MATLAB Function  TreatAsAtomicUnit=on
  Delayed : Outport
  wires:
  Bus Selector/3 -> Mux4/3  "<rudder>"
  Bus Selector/2 -> Mux4/2  "<elevator>"
  Bus Selector/1 -> Mux4/1  "<aileron>"
  Switch1/1 -> Demux/1
  Safety_Switch/1 -> Switch1/2
  RC_controls/1 -> Switch1/1
  Demux/4 -> limit control output3/1(u), Scope1/4
  Bus Selector/4 -> Mux4/4  "<thrust>"
  MATLAB Function1/1(out) -> Switch1/3
  limit control output/1(y) -> cmd2deg/2(u), Scope/2
  cmd2deg/1(y) -> act_alg/1, Scope/3
  Mux/1 -> limit control output/1(u), Scope/1
  Mux4/1 -> Scope2/1, MATLAB Function1/1(in)
  Data Type Conversion1/1 -> Delayed/1
  AP_controls/1 -> Bus Selector/1
  Demux/2 -> Mux/2
  Demux/1 -> Mux/1
  Demux/3 -> Mux/3
  act_alg/1 -> Mux1/1, Scope/4
  Mux1/1 -> Data Type Conversion1/1
  act_lims/1 -> cmd2deg/1(act_limits)
  limit control output3/1(y) -> Scope1/3, act_alg2/1, Scope1/2
  act_alg2/1 -> Mux1/2, Scope1/1

== system gnc_simplified/Subsystem/Actuator_Model/Subsystem1 ==
  note: [ Aileron	  ]
      | [ Elevator ]
      | [ Rudder	  ]
      | [ Thrust	  ]
  note: Signal Limits:
      | Aileron		[-1, 1]
      | Elevator		[-1, 1]
      | Rudder		[-1, 1]
      | Thrust		[0, 1]
  note: (1) test_controls
      | (2) steady_state
      | (3) wp_tracking
  note: Input from Gram RC:
      | 1 Thrust
      | 2 Aileron right
      | 3 Aileron left
      | 4 Flaperon right
      | 5 Flaperon left
      | 6 Elevator right
      | 7 Elevator left
      | 8 Gear
      | 9 Safety
      | 10 Arming
      | 11 Mode switch
      | 12 Elevator clean
      | 13 Rudder clean
      | 16 Aileron clean
  RC_channels : Inport  OutDataTypeStr=Bus: IFRCG_Bus_Topic_RcChannels
  Bus Selector1 : BusSelector  OutputSignals=channels
  Demux1 : Demux  Outputs=6
  MATLAB Function : MATLAB Function  TreatAsAtomicUnit=on
  Mux : Mux
  Scope : Scope  NumInputPorts=2
      settings: ActiveDisplayYMinimum=-1.5  ActiveDisplayYMaximum=3.5  DataLoggingVariableName=ScopeData3
  Scope1 : Scope
      settings: ActiveDisplayYMinimum=-1.5  ActiveDisplayYMaximum=3.5  DataLoggingVariableName=ScopeData7
  Selector : Selector  InputPortWidth=18  IndexOptions=Index vector (dialog)  Indices=[16 12 13 1 11 9]  OutputSizes=1
  rc_mode : Outport  OutDataTypeStr=uint8
  RC_controls : Outport  Port=2
  Safety_Switch : Outport  Port=3
  wires:
  Bus Selector1/1 -> Selector/1  "<channels>"
  Demux1/4 -> Mux/4
  Demux1/6 -> Scope1/1, Safety_Switch/1
  RC_channels/1 -> Bus Selector1/1
  Demux1/5 -> Scope/2, MATLAB Function/1(u)
  Mux/1 -> RC_controls/1
  Selector/1 -> Demux1/1
  MATLAB Function/1(y) -> rc_mode/1, Scope/1
  Demux1/2 -> Mux/2
  Demux1/1 -> Mux/1
  Demux1/3 -> Mux/3

== system gnc_simplified/Subsystem/Subsystem1/codegen_topic_publication ==
  publish_topic : Inport  OutDataTypeStr=boolean
  Bus_Creator : BusCreator  Inputs=1  OutDataTypeStr=Bus: IFRCG_Bus_CodeGenInternalTopicPublication
      settings: InheritFromInputs=off
  bus_codegen_topic_publication : Outport  OutDataTypeStr=Bus: IFRCG_Bus_CodeGenInternalTopicPublication
  wires:
  publish_topic/1 -> Bus_Creator/1
  Bus_Creator/1 -> bus_codegen_topic_publication/1

== system gnc_simplified/Subsystem/Subsystem1/codegen_topic_subscription ==
  Bus_Creator : BusCreator  Inputs=2  OutDataTypeStr=Bus: IFRCG_Bus_CodeGenInternalTopicSubscription
      settings: InheritFromInputs=off
  updated : Constant  Value=false  OutDataTypeStr=boolean
  updated_counter : Constant  Value=0  OutDataTypeStr=uint64
  bus_codegen_topic_subscription : Outport  OutDataTypeStr=Bus: IFRCG_Bus_CodeGenInternalTopicSubscription
  wires:
  Bus_Creator/1 -> bus_codegen_topic_subscription/1
  updated_counter/1 -> Bus_Creator/2
  updated/1 -> Bus_Creator/1
